simulink model "ARsim"  (R2022b)
settings: Solver=VariableStepAuto  StartTime=0.0  StopTime=10.0  RelTol=1e-3
undefined symbols (not defined in the file): b_p, J, K_e, K_hat_e, K_t, K_v, L_p, R_a, R_hat_p, R_p
settings Model: Creator=qingchuanhou  LastModifiedBy=qingchuanhou

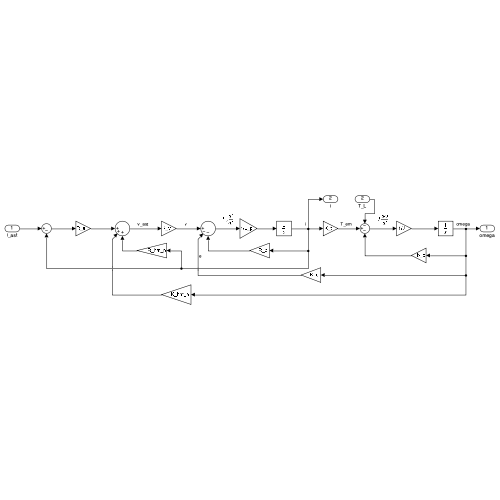
[thumbnail: Simulink's stored preview of the top-level diagram]
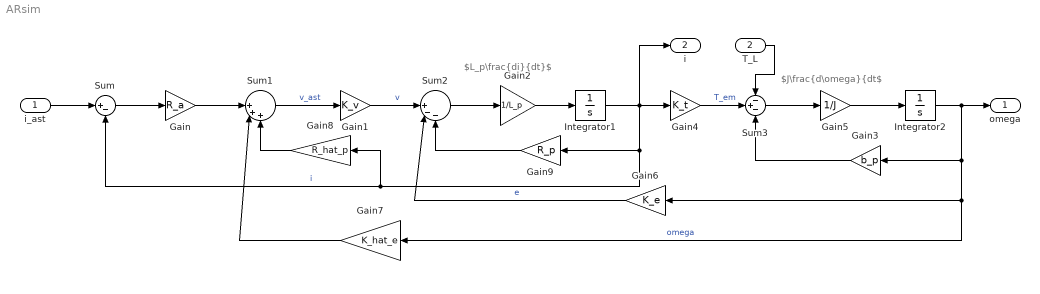
== system ARsim ==
  note: $J\frac{d\omega}{dt$
  note: $L_p\frac{di}{dt}$
  i_ast : Inport
  T_L : Inport  Port=2
  Gain : Gain  Gain=R_a
  Gain1 : Gain  Gain=K_v
  Gain2 : Gain  Gain=1/L_p
  Gain3 : Gain  Gain=b_p
  Gain4 : Gain  Gain=K_t
  Gain5 : Gain  Gain=1/J
  Gain6 : Gain  Gain=K_e
  Gain7 : Gain  Gain=K_hat_e
  Gain8 : Gain  Gain=R_hat_p
  Gain9 : Gain  Gain=R_p
  Integrator1 : Integrator
  Integrator2 : Integrator
  Sum : Sum  Inputs=|+-
  Sum1 : Sum  Inputs=||+++
  Sum2 : Sum  Inputs=||+--
  Sum3 : Sum  Inputs=-+-
  omega : Outport
  i : Outport  Port=2
  wires:
  Sum/1 -> Gain/1
  Gain/1 -> Sum1/1
  Sum1/1 -> Gain1/1  "v_ast"
  Gain1/1 -> Sum2/1  "v"
  Sum2/1 -> Gain2/1
  Gain2/1 -> Integrator1/1
  Integrator1/1 -> Gain4/1, i/1, Gain9/1, Sum/2, Gain8/1  "i"
  Gain4/1 -> Sum3/2  "T_em"
  Sum3/1 -> Gain5/1
  Gain5/1 -> Integrator2/1
  i_ast/1 -> Sum/1
  Integrator2/1 -> Gain7/1, Gain6/1, Gain3/1, omega/1  "omega"
  Gain3/1 -> Sum3/3
  Gain6/1 -> Sum2/2  "e"
  Gain7/1 -> Sum1/2
  Gain9/1 -> Sum2/3
  T_L/1 -> Sum3/1
  Gain8/1 -> Sum1/3
